simulink model "model2014a"  (R2014a)
settings: Solver=ode4  StartTime=0.0  StopTime=10  FixedStep=0.001  RelTol=1e-3
undefined symbols (not defined in the file): params
libraries: simulink x2
settings Model: Creator=Edo  LastModifiedBy=jelavice
settings DebuggingCC: MergeDetectMultiDrivingBlocksExec=error  FrameProcessingCompatibilityMsg=error

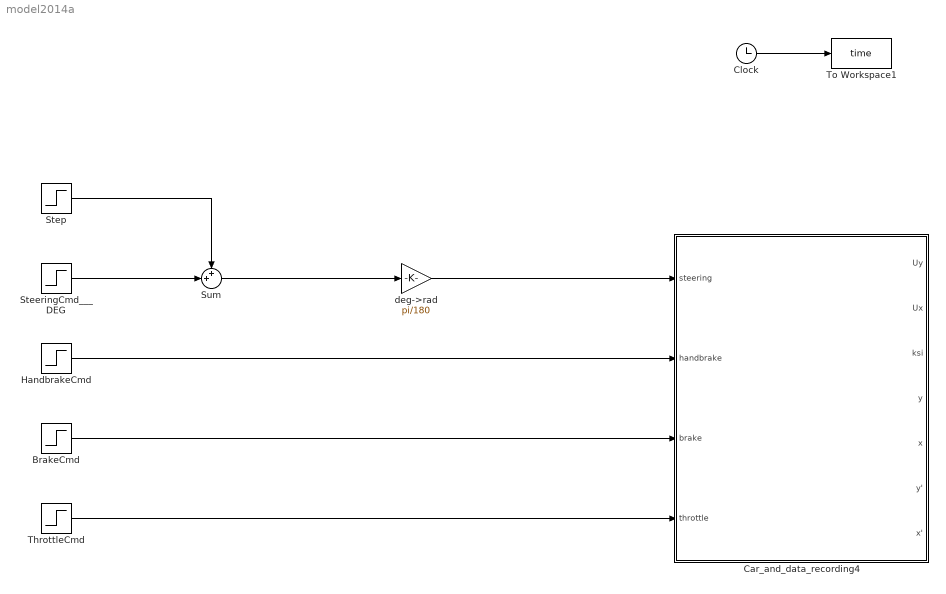
== system model2014a ==
  BrakeCmd : Step  Time=2  After=0  SampleTime=0
  Car_and_data_recording4 : Subsystem
  Clock : Clock
  HandbrakeCmd : Step  Time=3.2  SampleTime=0
  SteeringCmd___DEG : Step  Time=3  After=15  SampleTime=0
  Step : Step  After=0  SampleTime=0
  Sum : Sum  Inputs=++|
  ThrottleCmd : Step  Time=0.1  After=0  SampleTime=0
  To Workspace1 : ToWorkspace  VariableName=time  SampleTime=-1
  deg->rad : Gain  Gain=pi/180
  wires:
  Clock/1 -> To Workspace1/1
  SteeringCmd___DEG/1 -> Sum/2
  Step/1 -> Sum/1
  deg->rad/1 -> Car_and_data_recording4/1(steering)
  BrakeCmd/1 -> Car_and_data_recording4/3(brake)
  HandbrakeCmd/1 -> Car_and_data_recording4/2(handbrake)
  ThrottleCmd/1 -> Car_and_data_recording4/4(throttle)
  Sum/1 -> deg->rad/1

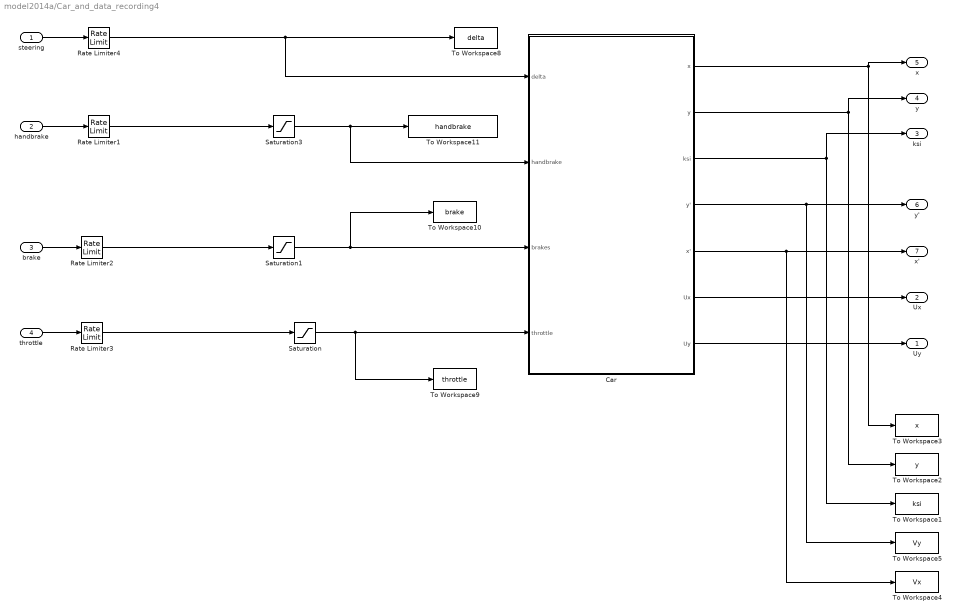
== system model2014a/Car_and_data_recording4 ==
  steering : Inport
  handbrake : Inport  Port=2
  brake : Inport  Port=3
  throttle : Inport  Port=4
  Car : Subsystem
  Rate Limiter1 : RateLimiter  RisingSlewLimit=5  FallingSlewLimit=-5  SampleTimeMode=inherited
  Rate Limiter2 : RateLimiter  RisingSlewLimit=5  FallingSlewLimit=-5  SampleTimeMode=inherited
  Rate Limiter3 : RateLimiter  RisingSlewLimit=5  FallingSlewLimit=-5  SampleTimeMode=inherited
  Rate Limiter4 : RateLimiter  RisingSlewLimit=50*pi/180  FallingSlewLimit=-50*pi/180  SampleTimeMode=inherited
  Saturation : Saturate  UpperLimit=1  LowerLimit=0
  Saturation1 : Saturate  UpperLimit=1  LowerLimit=0
  Saturation3 : Saturate  UpperLimit=1  LowerLimit=0
  To Workspace1 : ToWorkspace  VariableName=ksi  SampleTime=-1
  To Workspace10 : ToWorkspace  VariableName=brake  SampleTime=-1
  To Workspace11 : ToWorkspace  VariableName=handbrake  SampleTime=-1
  To Workspace2 : ToWorkspace  VariableName=y  SampleTime=-1
  To Workspace3 : ToWorkspace  VariableName=x  SampleTime=-1
  To Workspace4 : ToWorkspace  VariableName=Vx  SampleTime=-1
  To Workspace5 : ToWorkspace  VariableName=Vy  SampleTime=-1
  To Workspace8 : ToWorkspace  VariableName=delta  SampleTime=-1
  To Workspace9 : ToWorkspace  VariableName=throttle  SampleTime=-1
  Uy : Outport
  Ux : Outport  Port=2
  ksi : Outport  Port=3
  y : Outport  Port=4
  x : Outport  Port=5
  y' : Outport  Port=6
  x' : Outport  Port=7
  wires:
  Car/3(ksi) -> ksi/1, To Workspace1/1
  Car/2(y) -> y/1, To Workspace2/1
  Car/1(x) -> x/1, To Workspace3/1
  Car/4(y') -> y'/1, To Workspace5/1
  Saturation/1 -> Car/4(throttle), To Workspace9/1
  Saturation1/1 -> Car/3(brakes), To Workspace10/1
  steering/1 -> Rate Limiter4/1
  handbrake/1 -> Rate Limiter1/1
  brake/1 -> Rate Limiter2/1
  Car/5(x') -> x'/1, To Workspace4/1
  Saturation3/1 -> To Workspace11/1, Car/2(handbrake)
  throttle/1 -> Rate Limiter3/1
  Car/6(Ux) -> Ux/1
  Car/7(Uy) -> Uy/1
  Rate Limiter1/1 -> Saturation3/1
  Rate Limiter2/1 -> Saturation1/1
  Rate Limiter3/1 -> Saturation/1
  Rate Limiter4/1 -> To Workspace8/1, Car/1(delta)

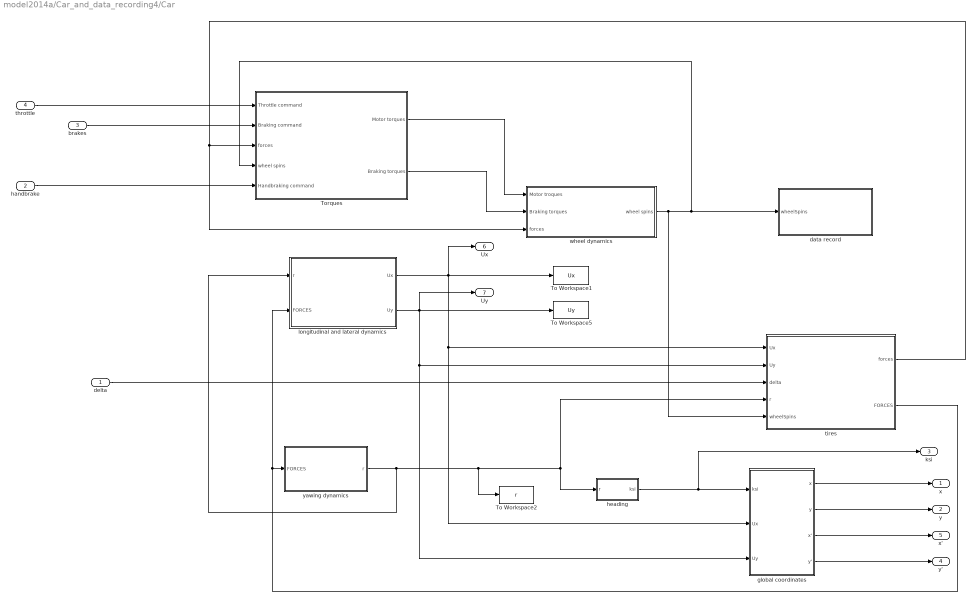
== system model2014a/Car_and_data_recording4/Car ==
  delta : Inport
  handbrake : Inport  Port=2
  brakes : Inport  Port=3
  throttle : Inport  Port=4
  To Workspace1 : ToWorkspace  VariableName=Ux  SampleTime=-1
  To Workspace2 : ToWorkspace  VariableName=r  SampleTime=-1
  To Workspace5 : ToWorkspace  VariableName=Uy  SampleTime=-1
  Torques : Subsystem
  data record : Subsystem
  global coordinates : Subsystem
  "heading " : Subsystem
  longitudinal and lateral dynamics : Subsystem
  tires : Subsystem
  wheel dynamics : Subsystem
  yawing dynamics : Subsystem
  x : Outport
  y : Outport  Port=2
  ksi : Outport  Port=3
  y' : Outport  Port=4
  x' : Outport  Port=5
  Ux : Outport  Port=6
  Uy : Outport  Port=7
  wires:
  Torques/1(Motor torques) -> wheel dynamics/1(Motor troques)
  Torques/2(Braking torques) -> wheel dynamics/2(Braking torques)
  yawing dynamics/1(r) -> longitudinal and lateral dynamics/1(r), To Workspace2/1, tires/4(r), "heading "/1(r)
  longitudinal and lateral dynamics/1(Ux) -> Ux/1, To Workspace1/1, global coordinates/2(Ux), tires/1(Ux)
  longitudinal and lateral dynamics/2(Uy) -> Uy/1, To Workspace5/1, global coordinates/3(Uy), tires/2(Uy)
  global coordinates/1(x) -> x/1
  global coordinates/2(y) -> y/1
  handbrake/1 -> Torques/5(Handbraking command)
  brakes/1 -> Torques/2(Braking command)
  throttle/1 -> Torques/1(Throttle command)
  delta/1 -> tires/3(delta)
  "heading "/1(ksi) -> ksi/1, global coordinates/1(ksi)
  global coordinates/4(y') -> y'/1
  global coordinates/3(x') -> x'/1
  wheel dynamics/1(wheel spins) -> tires/5(wheelSpins), data record/1(wheelSpins), Torques/4(wheel spins)
  tires/2(FORCES) -> yawing dynamics/1(FORCES), longitudinal and lateral dynamics/2(FORCES)
  tires/1(forces) -> wheel dynamics/3(forces), Torques/3(forces)

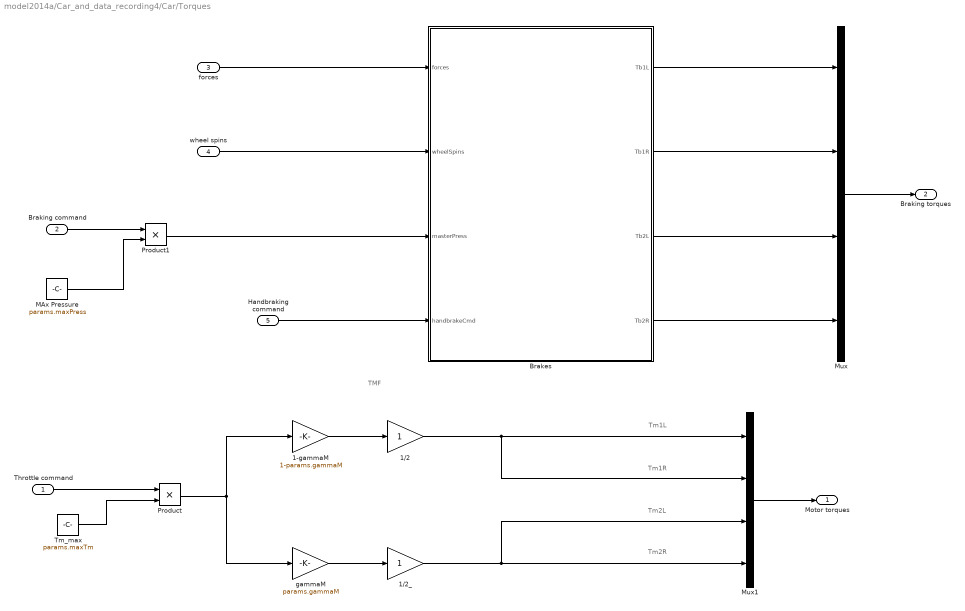
== system model2014a/Car_and_data_recording4/Car/Torques ==
  note: Tm2R
  note: Tm2L
  note: Tm1R
  note: Tm1L
  note: TMF
  Throttle command : Inport
  Braking command : Inport  Port=2
  forces : Inport  Port=3
  wheel spins : Inport  Port=4
  Handbraking command : Inport  Port=5
  1-gammaM : Gain  Gain=1-params.gammaM
  1/2 : Gain
  1/2_ : Gain
  Brakes : MATLAB Function  TreatAsAtomicUnit=on
      settings: PermitHierarchicalResolution=ParametersOnly
  MAx Pressure : Constant  Value=params.maxPress
  Mux : Mux
  Mux1 : Mux
  Product : Product
  Product1 : Product
  Tm_max : Constant  Value=params.maxTm
  gammaM : Gain  Gain=params.gammaM
  Motor torques : Outport
  Braking torques : Outport  Port=2
  wires:
  Throttle command/1 -> Product/1
  Tm_max/1 -> Product/2
  MAx Pressure/1 -> Product1/2
  Braking command/1 -> Product1/1
  Brakes/1(Tb1L) -> Mux/1
  Brakes/2(Tb1R) -> Mux/2
  Mux/1 -> Braking torques/1
  Mux1/1 -> Motor torques/1
  Product/1 -> 1-gammaM/1, gammaM/1
  wheel spins/1 -> Brakes/2(wheelSpins)
  Product1/1 -> Brakes/3(masterPress)
  Handbraking command/1 -> Brakes/4(handbrakeCmd)
  forces/1 -> Brakes/1(forces)
  Brakes/3(Tb2L) -> Mux/3
  Brakes/4(Tb2R) -> Mux/4
  1-gammaM/1 -> 1/2/1
  gammaM/1 -> 1/2_/1
  1/2/1 -> Mux1/2, Mux1/1
  1/2_/1 -> Mux1/4, Mux1/3

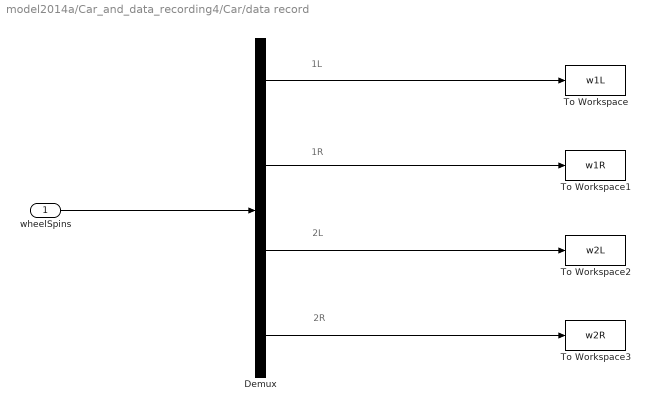
== system model2014a/Car_and_data_recording4/Car/data record ==
  note: 2R
  note: 2L
  note: 1R
  note: 1L
  wheelSpins : Inport
  Demux : Demux
  To Workspace : ToWorkspace  VariableName=w1L  SampleTime=-1
  To Workspace1 : ToWorkspace  VariableName=w1R  SampleTime=-1
  To Workspace2 : ToWorkspace  VariableName=w2L  SampleTime=-1
  To Workspace3 : ToWorkspace  VariableName=w2R  SampleTime=-1
  wires:
  Demux/1 -> To Workspace/1
  Demux/2 -> To Workspace1/1
  Demux/3 -> To Workspace2/1
  Demux/4 -> To Workspace3/1
  wheelSpins/1 -> Demux/1

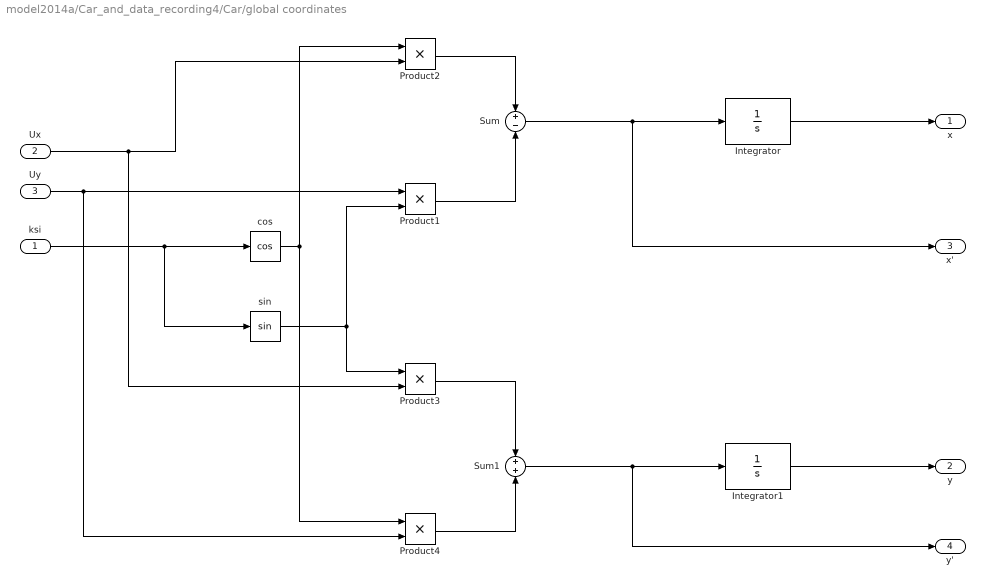
== system model2014a/Car_and_data_recording4/Car/global coordinates ==
  ksi : Inport
  Ux : Inport  Port=2
  Uy : Inport  Port=3
  Integrator : Integrator  InitialCondition=params.x0
  Integrator1 : Integrator  InitialCondition=params.y0
  Product{1..4} (4 alike) : Product
  Sum : Sum  Inputs=+|-
  Sum1 : Sum  Inputs=+|+
  cos : Trigonometry  Operator=cos
  sin : Trigonometry
  x : Outport
  y : Outport  Port=2
  x' : Outport  Port=3
  y' : Outport  Port=4
  wires:
  Integrator/1 -> x/1
  ksi/1 -> sin/1, cos/1
  cos/1 -> Product4/1, Product2/1
  Integrator1/1 -> y/1
  Ux/1 -> Product3/2, Product2/2
  Product2/1 -> Sum/1
  Sum/1 -> x'/1, Integrator/1
  Product1/1 -> Sum/2
  Uy/1 -> Product4/2, Product1/1
  sin/1 -> Product3/1, Product1/2
  Product3/1 -> Sum1/1
  Product4/1 -> Sum1/2
  Sum1/1 -> y'/1, Integrator1/1

== system model2014a/Car_and_data_recording4/Car/heading  ==
  r : Inport
  Integrator : Integrator  InitialCondition=params.ksi0
  ksi : Outport
  wires:
  Integrator/1 -> ksi/1
  r/1 -> Integrator/1

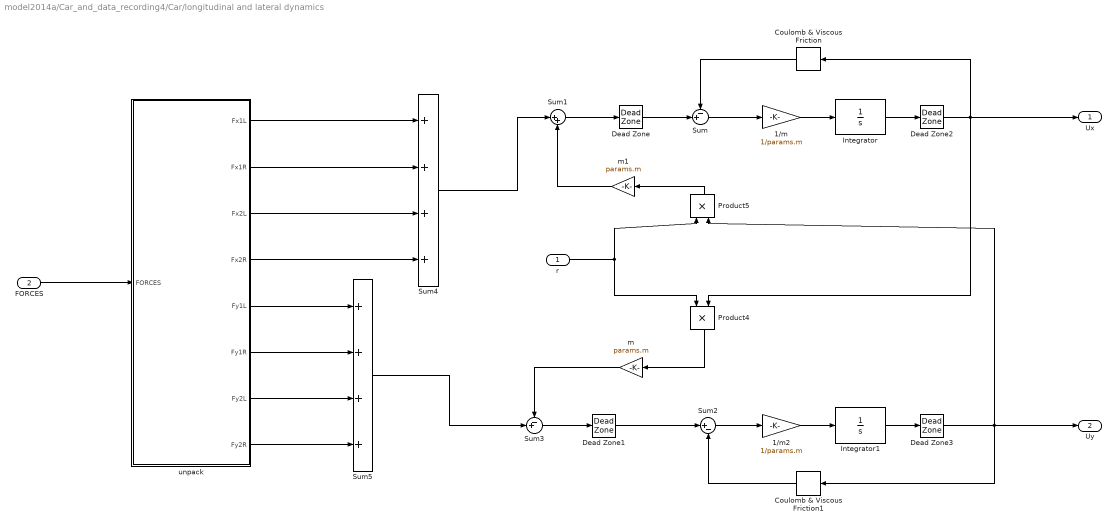
== system model2014a/Car_and_data_recording4/Car/longitudinal and lateral dynamics ==
  r : Inport
  FORCES : Inport  Port=2
  1/m : Gain  Gain=1/params.m
  1/m2 : Gain  Gain=1/params.m
  Coulomb & Viscous Friction : simulink/Discontinuities/Coulomb & Viscous Friction  offset=params.fric  gain=params.b
  Coulomb & Viscous Friction1 : simulink/Discontinuities/Coulomb & Viscous Friction  offset=params.fric*0  gain=params.b*0
  Dead Zone : DeadZone  LowerValue=-params.m*params.g*params.muRoll  UpperValue=params.m*params.g*params.muRoll  SaturateOnIntegerOverflow=on
  Dead Zone1 : DeadZone  LowerValue=-params.m*params.g*params.muRoll  UpperValue=params.m*params.g*params.muRoll  SaturateOnIntegerOverflow=on
  Dead Zone2 : DeadZone  LowerValue=-params.Dz1  UpperValue=params.Dz1  SaturateOnIntegerOverflow=on
  Dead Zone3 : DeadZone  LowerValue=-params.Dz1  UpperValue=params.Dz1  SaturateOnIntegerOverflow=on
  Integrator : Integrator  InitialCondition=params.Ux0
  Integrator1 : Integrator  InitialCondition=params.Uy0
  Product4 : Product
  Product5 : Product
  Sum : Sum  Inputs=-+|
  Sum1 : Sum  Inputs=|++
  Sum2 : Sum  Inputs=|+-
  Sum3 : Sum  Inputs=-+|
  Sum4 : Sum  Inputs=++++
  Sum5 : Sum  Inputs=++++
  m : Gain  Gain=params.m
  m1 : Gain  Gain=params.m
  unpack : Subsystem
  Ux : Outport
  Uy : Outport  Port=2
  wires:
  Sum2/1 -> 1/m2/1
  Product4/1 -> m/1
  r/1 -> Product5/1, Product4/1
  Integrator1/1 -> Dead Zone3/1
  Integrator/1 -> Dead Zone2/1
  Dead Zone1/1 -> Sum2/1
  1/m2/1 -> Integrator1/1
  m/1 -> Sum3/1
  Sum3/1 -> Dead Zone1/1
  Sum5/1 -> Sum3/2
  1/m/1 -> Integrator/1
  Sum4/1 -> Sum1/1
  Sum1/1 -> Dead Zone/1
  Product5/1 -> m1/1
  Dead Zone/1 -> Sum/2
  Sum/1 -> 1/m/1
  Coulomb & Viscous Friction/1 -> Sum/1
  m1/1 -> Sum1/2
  Dead Zone2/1 -> Coulomb & Viscous Friction/1, Ux/1, Product4/2
  Dead Zone3/1 -> Coulomb & Viscous Friction1/1, Uy/1, Product5/2
  FORCES/1 -> unpack/1(FORCES)
  unpack/1(Fx1L) -> Sum4/1
  unpack/2(Fx1R) -> Sum4/2
  unpack/3(Fx2L) -> Sum4/3
  unpack/4(Fx2R) -> Sum4/4
  unpack/5(Fy1L) -> Sum5/1
  unpack/6(Fy1R) -> Sum5/2
  unpack/7(Fy2L) -> Sum5/3
  unpack/8(Fy2R) -> Sum5/4
  Coulomb & Viscous Friction1/1 -> Sum2/2

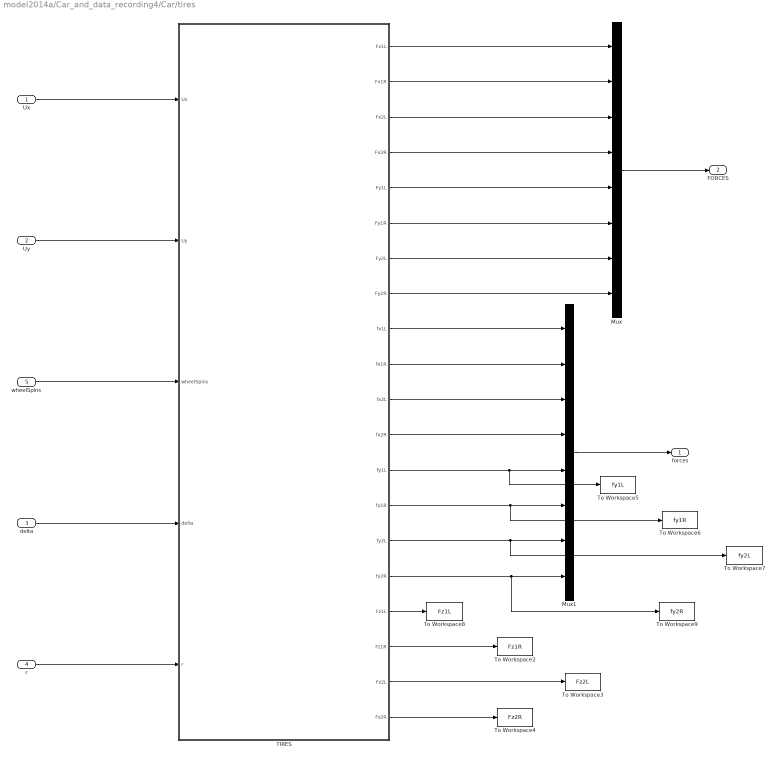
== system model2014a/Car_and_data_recording4/Car/tires ==
  Ux : Inport
  Uy : Inport  Port=2
  delta : Inport  Port=3
  r : Inport  Port=4
  wheelSpins : Inport  Port=5
  Mux : Mux  Inputs=8
  Mux1 : Mux  Inputs=8
  TIRES : MATLAB Function  TreatAsAtomicUnit=on
      settings: PermitHierarchicalResolution=ParametersOnly
  To Workspace2 : ToWorkspace  VariableName=Fz1R  SampleTime=-1
  To Workspace3 : ToWorkspace  VariableName=Fz2L  SampleTime=-1
  To Workspace4 : ToWorkspace  VariableName=Fz2R  SampleTime=-1
  To Workspace5 : ToWorkspace  VariableName=fy1L  SampleTime=-1
  To Workspace6 : ToWorkspace  VariableName=fy1R  SampleTime=-1
  To Workspace7 : ToWorkspace  VariableName=fy2L  SampleTime=-1
  To Workspace8 : ToWorkspace  VariableName=Fz1L  SampleTime=-1
  To Workspace9 : ToWorkspace  VariableName=fy2R  SampleTime=-1
  forces : Outport
  FORCES : Outport  Port=2
  wires:
  Ux/1 -> TIRES/1(Ux)
  Uy/1 -> TIRES/2(Uy)
  delta/1 -> TIRES/4(delta)
  r/1 -> TIRES/5(r)
  Mux/1 -> FORCES/1
  TIRES/1(Fx1L) -> Mux/1
  TIRES/2(Fx1R) -> Mux/2
  TIRES/3(Fx2L) -> Mux/3
  TIRES/4(Fx2R) -> Mux/4
  TIRES/5(Fy1L) -> Mux/5
  TIRES/6(Fy1R) -> Mux/6
  TIRES/7(Fy2L) -> Mux/7
  TIRES/8(Fy2R) -> Mux/8
  wheelSpins/1 -> TIRES/3(wheelSpins)
  TIRES/9(fx1L) -> Mux1/1
  TIRES/14(fy1R) -> To Workspace6/1, Mux1/6
  TIRES/10(fx1R) -> Mux1/2
  TIRES/13(fy1L) -> To Workspace5/1, Mux1/5
  TIRES/11(fx2L) -> Mux1/3
  TIRES/12(fx2R) -> Mux1/4
  TIRES/16(fy2R) -> To Workspace9/1, Mux1/8
  Mux1/1 -> forces/1
  TIRES/17(Fz1L) -> To Workspace8/1
  TIRES/18(Fz1R) -> To Workspace2/1
  TIRES/19(Fz2L) -> To Workspace3/1
  TIRES/20(Fz2R) -> To Workspace4/1
  TIRES/15(fy2L) -> To Workspace7/1, Mux1/7

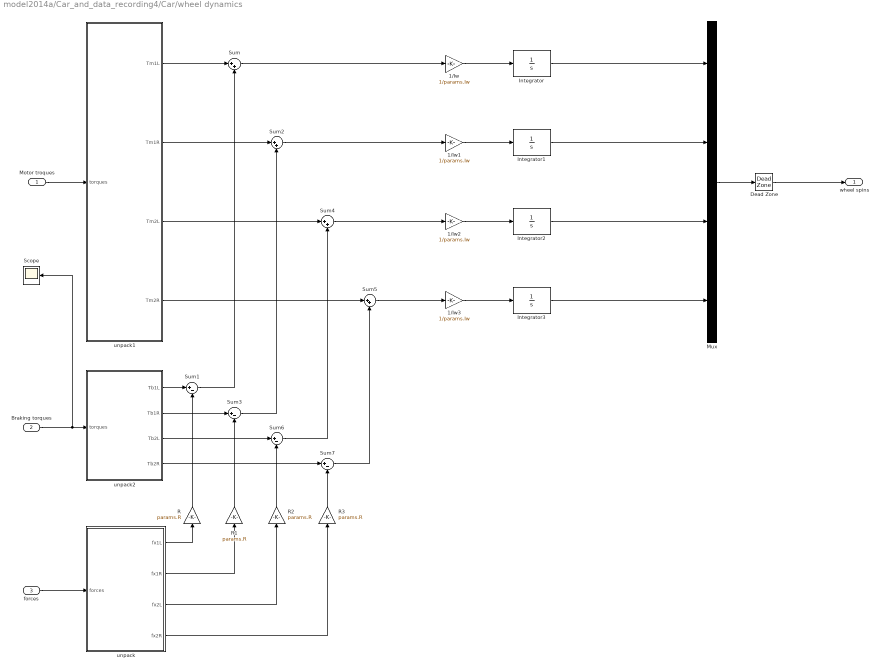
== system model2014a/Car_and_data_recording4/Car/wheel dynamics ==
  Motor troques : Inport
  Braking torques : Inport  Port=2
  forces : Inport  Port=3
  1/Iw{,1..3} (4 alike) : Gain  Gain=1/params.Iw
  Dead Zone : DeadZone  LowerValue=-params.Dz1/params.R  UpperValue=params.Dz1/params.R  SaturateOnIntegerOverflow=on
  Integrator : Integrator  InitialCondition=params.w1L0  LimitOutput=on  LowerSaturationLimit=0
  Integrator1 : Integrator  InitialCondition=params.w1R0  LimitOutput=on  LowerSaturationLimit=0
  Integrator2 : Integrator  InitialCondition=params.w2L0  LimitOutput=on  LowerSaturationLimit=0
  Integrator3 : Integrator  InitialCondition=params.w2R0  LimitOutput=on  LowerSaturationLimit=0
  Mux : Mux
  R{,1..3} (4 alike) : Gain  Gain=params.R
  Scope : Scope
      settings: TimeRange=auto  MaxDataPoints=5000  SaveToWorkspace=off  SaveName=ScopeData  YMin=-10  YMax=10  SampleTime=-1  DataFormat=Array
  Sum{,2,4..5} (4 alike) : Sum  Inputs=|++
  Sum{1,3,6..7} (4 alike) : Sum  Inputs=|+-
  unpack : Subsystem
  unpack1 : Subsystem
  unpack2 : Subsystem
  wheel spins : Outport  PortDimensions=4
  wires:
  1/Iw/1 -> Integrator/1
  1/Iw1/1 -> Integrator1/1
  forces/1 -> unpack/1(forces)
  Motor troques/1 -> unpack1/1(torques)
  Braking torques/1 -> Scope/1, unpack2/1(torques)
  unpack1/1(Tm1L) -> Sum/1
  unpack/1(fx1L) -> R/1
  unpack2/1(Tb1L) -> Sum1/1
  Sum1/1 -> Sum/2
  Sum/1 -> 1/Iw/1
  unpack1/2(Tm1R) -> Sum2/1
  unpack2/2(Tb1R) -> Sum3/1
  unpack/2(fx1R) -> R1/1
  Sum3/1 -> Sum2/2
  Sum2/1 -> 1/Iw1/1
  1/Iw2/1 -> Integrator2/1
  unpack1/3(Tm2L) -> Sum4/1
  Sum4/1 -> 1/Iw2/1
  unpack1/4(Tm2R) -> Sum5/1
  1/Iw3/1 -> Integrator3/1
  Sum5/1 -> 1/Iw3/1
  unpack2/3(Tb2L) -> Sum6/1
  unpack/3(fx2L) -> R2/1
  Sum6/1 -> Sum4/2
  unpack2/4(Tb2R) -> Sum7/1
  unpack/4(fx2R) -> R3/1
  Sum7/1 -> Sum5/2
  R/1 -> Sum1/2
  R1/1 -> Sum3/2
  R2/1 -> Sum6/2
  R3/1 -> Sum7/2
  Mux/1 -> Dead Zone/1
  Integrator/1 -> Mux/1
  Integrator1/1 -> Mux/2
  Integrator2/1 -> Mux/3
  Integrator3/1 -> Mux/4
  Dead Zone/1 -> wheel spins/1

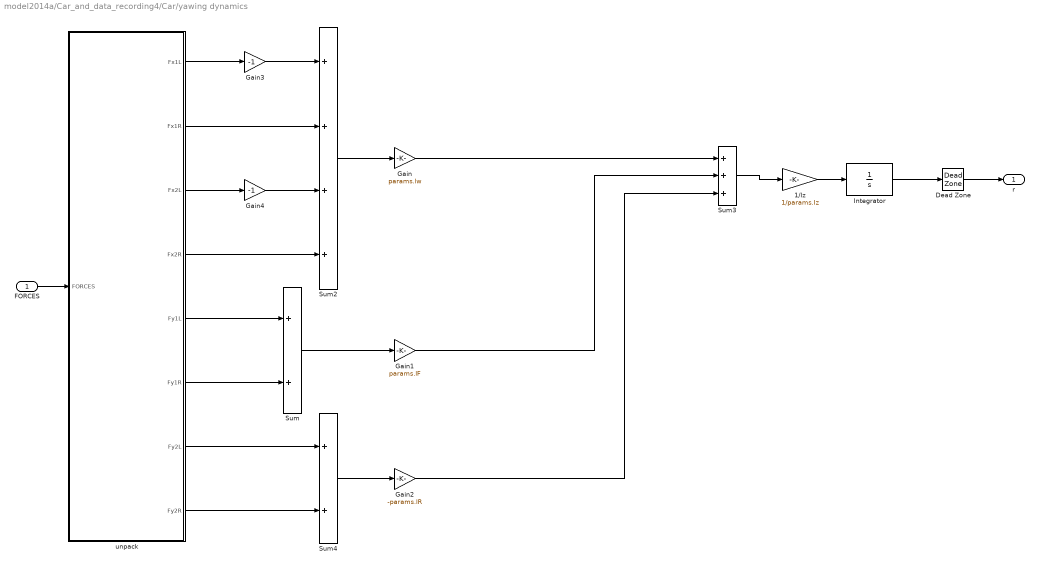
== system model2014a/Car_and_data_recording4/Car/yawing dynamics ==
  FORCES : Inport
  1/Iz : Gain  Gain=1/params.Iz
  Dead Zone : DeadZone  LowerValue=-params.Dz2  UpperValue=params.Dz2  SaturateOnIntegerOverflow=on
  Gain : Gain  Gain=params.lw
  Gain1 : Gain  Gain=params.lF
  Gain2 : Gain  Gain=-params.lR
  Gain3 : Gain  Gain=-1
  Gain4 : Gain  Gain=-1
  Integrator : Integrator  InitialCondition=params.r0
  Sum : Sum
  Sum2 : Sum  Inputs=++++
  Sum3 : Sum  Inputs=+++
  Sum4 : Sum
  unpack : Subsystem
  r : Outport
  wires:
  1/Iz/1 -> Integrator/1
  Sum3/1 -> 1/Iz/1
  Integrator/1 -> Dead Zone/1
  Dead Zone/1 -> r/1
  Sum2/1 -> Gain/1
  Sum4/1 -> Gain2/1
  Sum/1 -> Gain1/1
  unpack/2(Fx1R) -> Sum2/2
  unpack/4(Fx2R) -> Sum2/4
  Gain/1 -> Sum3/1
  Gain1/1 -> Sum3/2
  Gain2/1 -> Sum3/3
  FORCES/1 -> unpack/1(FORCES)
  unpack/1(Fx1L) -> Gain3/1
  unpack/3(Fx2L) -> Gain4/1
  unpack/5(Fy1L) -> Sum/1
  unpack/6(Fy1R) -> Sum/2
  unpack/7(Fy2L) -> Sum4/1
  unpack/8(Fy2R) -> Sum4/2
  Gain4/1 -> Sum2/3
  Gain3/1 -> Sum2/1

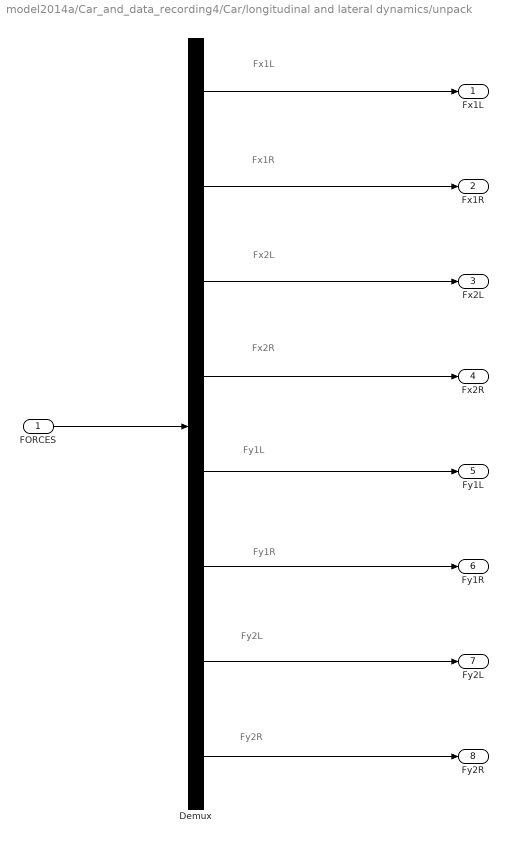
== system model2014a/Car_and_data_recording4/Car/longitudinal and lateral dynamics/unpack ==
  note: Fy2R
  note: Fy2L
  note: Fy1R
  note: Fy1L
  note: Fx2R
  note: Fx2L
  note: Fx1R
  note: Fx1L
  FORCES : Inport
  Demux : Demux  Outputs=8
  Fx1L : Outport
  Fx1R : Outport  Port=2
  Fx2L : Outport  Port=3
  Fx2R : Outport  Port=4
  Fy1L : Outport  Port=5
  Fy1R : Outport  Port=6
  Fy2L : Outport  Port=7
  Fy2R : Outport  Port=8
  wires:
  FORCES/1 -> Demux/1
  Demux/2 -> Fx1R/1
  Demux/4 -> Fx2R/1
  Demux/6 -> Fy1R/1
  Demux/5 -> Fy1L/1
  Demux/1 -> Fx1L/1
  Demux/3 -> Fx2L/1
  Demux/7 -> Fy2L/1
  Demux/8 -> Fy2R/1

== system model2014a/Car_and_data_recording4/Car/wheel dynamics/unpack ==
  note: Fy2R
  note: Fy2L
  note: Fy1R
  note: Fy1L
  note: Fx2R
  note: Fx2L
  note: Fx1R
  note: Fx1L
  forces : Inport
  Demux : Demux  Outputs=8
  fx1L : Outport
  fx1R : Outport  Port=2
  fx2L : Outport  Port=3
  fx2R : Outport  Port=4
  wires:
  forces/1 -> Demux/1
  Demux/1 -> fx1L/1
  Demux/4 -> fx2R/1
  Demux/3 -> fx2L/1
  Demux/2 -> fx1R/1

== system model2014a/Car_and_data_recording4/Car/wheel dynamics/unpack1 ==
  note: Tm2R
  note: Tm2L
  note: Tm1L
  note: Tm1R
  torques : Inport
  Demux1 : Demux
  Tm1L : Outport
  Tm1R : Outport  Port=2
  Tm2L : Outport  Port=3
  Tm2R : Outport  Port=4
  wires:
  torques/1 -> Demux1/1
  Demux1/1 -> Tm1L/1
  Demux1/2 -> Tm1R/1
  Demux1/4 -> Tm2R/1
  Demux1/3 -> Tm2L/1

== system model2014a/Car_and_data_recording4/Car/wheel dynamics/unpack2 ==
  note: Tb2R
  note: Tb2L
  note: Tb1L
  note: Tb1R
  torques : Inport
  Demux1 : Demux
  Tb1L : Outport
  Tb1R : Outport  Port=2
  Tb2L : Outport  Port=3
  Tb2R : Outport  Port=4
  wires:
  torques/1 -> Demux1/1
  Demux1/1 -> Tb1L/1
  Demux1/2 -> Tb1R/1
  Demux1/4 -> Tb2R/1
  Demux1/3 -> Tb2L/1

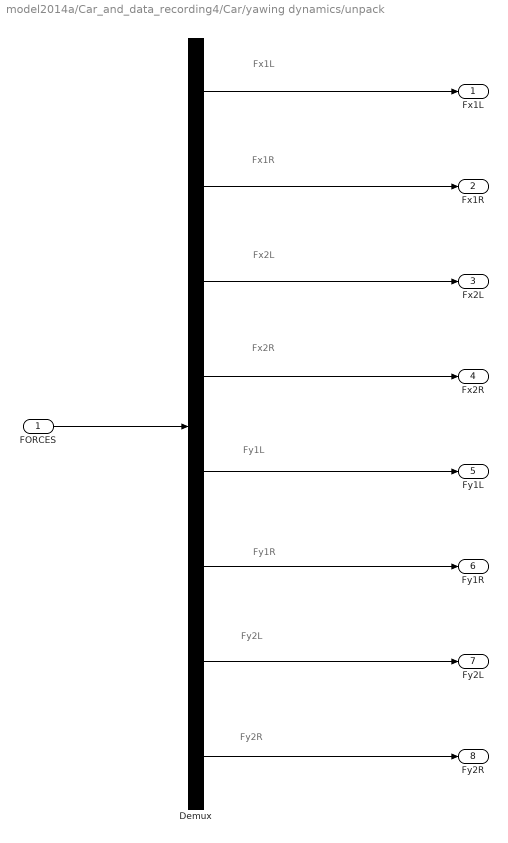
== system model2014a/Car_and_data_recording4/Car/yawing dynamics/unpack ==
  note: Fy2R
  note: Fy2L
  note: Fy1R
  note: Fy1L
  note: Fx2R
  note: Fx2L
  note: Fx1R
  note: Fx1L
  FORCES : Inport
  Demux : Demux  Outputs=8
  Fx1L : Outport
  Fx1R : Outport  Port=2
  Fx2L : Outport  Port=3
  Fx2R : Outport  Port=4
  Fy1L : Outport  Port=5
  Fy1R : Outport  Port=6
  Fy2L : Outport  Port=7
  Fy2R : Outport  Port=8
  wires:
  FORCES/1 -> Demux/1
  Demux/2 -> Fx1R/1
  Demux/4 -> Fx2R/1
  Demux/6 -> Fy1R/1
  Demux/5 -> Fy1L/1
  Demux/1 -> Fx1L/1
  Demux/3 -> Fx2L/1
  Demux/7 -> Fy2L/1
  Demux/8 -> Fy2R/1

== matlab function model2014a/Car_and_data_recording4/Car/Torques/Brakes ==
  data: forces input; Tb1L output; wheelSpins input; params parameter; masterPress input; handbrakeCmd input; Tb1R output; Tb2L output; Tb2R output
function [Tb1L, Tb1R, Tb2L, Tb2R] = brakes(forces,wheelSpins,params, masterPress, handbrakeCmd)
%#codegen

Tb1L = 0;
Tb1R = 0;
Tb2L = 0;
Tb2R = 0;

fx1L = forces(1);
fx1R = forces(2);
fx2L = forces(3);
fx2R = forces(4);

w1L = wheelSpins(1);
w1R = wheelSpins(2);
w2L = wheelSpins(3);
w2R = wheelSpins(4);

pressF = masterPress;
if masterPress <= 1.5
   pressR = masterPress; 
else
   pressR = 0.3 * masterPress + 1.05;
end
    
if masterPress > 0
   
    if w1L ~= 0
        Tb1L = - pressF * params.press2torF*sign(w1L);
    else
        Tb1L = fx1L * params.R;
    end
    
    if w1R ~= 0
        Tb1R = - pressF * params.press2torF*sign(w1R);
    else
        Tb1R = fx1R * params.R;
    end
    
    if w2L ~= 0
        Tb2L = Tb2L - pressR * params.press2torR*sign(w2L);
    else
        Tb2L = fx2L * params.R;
    end
    
    if w2R ~= 0
        Tb2R = Tb2R - pressR * params.press2torR*sign(w2R);
    else
        Tb2R = fx2R * params.R;
    end
end

if handbrakeCmd > 0
   
    if w2L ~= 0
        Tb2L = Tb2L - handbrakeCmd * params.maxThb*sign(w2L);
    else
        Tb2L = fx2L * params.R;
    end   
    
    if w2R ~= 0
        Tb2R = Tb2R - handbrakeCmd * params.maxThb*sign(w2R);
    else
        Tb2R = fx2R * params.R;
    end
end



end

== matlab function model2014a/Car_and_data_recording4/Car/tires/TIRES ==
  data: Ux input; Fx1L output; Uy input; wheelSpins input; delta input; r input; params parameter; Fx1R output; Fx2L output; Fx2R output; Fy1L output; Fy1R output; Fy2L output; Fy2R output; fx1L output; fx1R output; fx2L output; fx2R output; fy1L output; fy1R output; fy2L output; fy2R output; Fz1L output; Fz1R output; Fz2L output; Fz2R output
function [ Fx1L, Fx1R, Fx2L, Fx2R, Fy1L, Fy1R, Fy2L, Fy2R, fx1L, fx1R, fx2L, fx2R, fy1L, fy1R, fy2L, fy2R, Fz1L, Fz1R, Fz2L, Fz2R] = pacejka_model(Ux, Uy, wheelSpins, delta, r, params)
%#codegen

eps = 1e-4;

w1L = wheelSpins(1);
w1R = wheelSpins(2);
w2L = wheelSpins(3);
w2R = wheelSpins(4);

Ux1L = (Ux - r*params.lw)*cos(delta) + (Uy + r*params.lF)*sin(delta);
Uy1L = -(Ux - r*params.lw)*sin(delta) + (Uy + r*params.lF)*cos(delta);

Ux1R = (Ux + r*params.lw)*cos(delta) + (Uy + r*params.lF)*sin(delta);
Uy1R = -(Ux + r*params.lw)*sin(delta) + (Uy + r*params.lF)*cos(delta);

Ux2L = Ux - r*params.lw;
Uy2L = Uy - r*params.lR;

Ux2R = Ux + r*params.lw;
Uy2R = Uy - r*params.lR;


Sx1L = robustDiv2(Ux1L - params.R*w1L, params.R*w1L, eps);
Sy1L = (1+Sx1L) * robustDiv2(Uy1L, Ux1L, eps);

Sx1R = robustDiv2(Ux1R - params.R*w1R, params.R*w1R, eps);
Sy1R = (1+Sx1R) * robustDiv2(Uy1R, Ux1R, eps);

Sx2L = robustDiv2(Ux2L - params.R*w2L, params.R*w2L, eps);
Sy2L = (1+Sx2L) * robustDiv2(Uy2L, Ux2L, eps);

Sx2R = robustDiv2(Ux1R - params.R*w2R, params.R*w2R, eps);
Sy2R = (1+Sx2R) * robustDiv2(Uy2R, Ux2R, eps);



S1L = sqrt( (Sx1L)^2 + (Sy1L)^2 );
S1R = sqrt( (Sx1R)^2 + (Sy1R)^2 );
S2L = sqrt( (Sx2L)^2 + (Sy2L)^2 );
S2R = sqrt( (Sx2R)^2 + (Sy2R)^2 );

mu1L = params.D1*sin(params.C1*atan(params.B1*S1L));
mu1R = params.D1*sin(params.C1*atan(params.B1*S1R));
mu2L = params.D2*sin(params.C2*atan(params.B2*S2L));
mu2R = params.D2*sin(params.C2*atan(params.B2*S2R));

mux1L = - mu1L * robustDiv(Sx1L,S1L,eps);
muy1L = - mu1L * robustDiv(Sy1L,S1L,eps);

mux1R = - mu1R * robustDiv(Sx1R,S1R,eps);
muy1R = - mu1R * robustDiv(Sy1R,S1R,eps);

mux2L = - mu2L * robustDiv(Sx2L,S2L,eps);
muy2L = - mu2L * robustDiv(Sy2L,S2L,eps);

mux2R = - mu2R * robustDiv(Sx2R,S2R,eps);
muy2R = - mu2R * robustDiv(Sy2R,S2R,eps);



C1 = -params.mu*mux1L*params.h*sin(delta);
C2 = -params.mu*muy1L*params.h*cos(delta);
C3 = -params.mu*mux1R*params.h*sin(delta);
C4 = -params.mu*muy1R*params.h*cos(delta);
C5 = -params.mu*muy2L*params.h;
C6 = -params.mu*muy2R*params.h;
% 
K1 = params.mu*mux1L*params.h*cos(delta);
K2 = params.mu*muy1L*params.h*sin(delta);
K3 = params.mu*mux1R*params.h*cos(delta);
K4 = params.mu*muy1R*params.h*sin(delta);
K5 = params.mu*mux2L*params.h;
K6 = params.mu*mux2R*params.h;
% 
A = -params.lw - C1 - C2;
B = params.lw - C3 - C4;
C = -params.lw - C5;
D = params.lw - C6;
E = K1 - K2 - params.lF;
F = K3 - K4 - params.lF;
G = K5 + params.lR;
H = K6 + params.lR;

den = 2*(A*F - E*B - A*G + E*C + B*H - D*F - C*H + D*G);

Fz1L = params.m*params.g*(B*G - C*F + B*H - D*F - C*H + D*G)/den;
Fz1R = - params.m*params.g*(A*G - E*C + A*H - E*D + C*H - D*G)/den;
Fz2L = params.m*params.g*(A*F - E*B + A*H - E*D + B*H - D*F)/den;
Fz2R = params.m*params.g*(A*F - E*B - A*G + E*C - B*G + C*F)/den;


% Fz1L = 0.5* params.m*params.g * params.lR / (2.91);
% Fz1R = 0.5* params.m*params.g * params.lR / (2.91);
% Fz2L = 0.5* params.m*params.g * params.lF / (2.91);
% Fz2R = 0.5* params.m*params.g * params.lF / (2.91);



fx1L = params.mu*Fz1L*mux1L;
fy1L = params.mu*Fz1L*muy1L;

fx1R = params.mu*Fz1R*mux1R;
fy1R = params.mu*Fz1R*muy1R;

fx2L = params.mu*Fz2L*mux2L;
fy2L = params.mu*Fz2L*muy2L;

fx2R = params.mu*Fz2R*mux2R;
fy2R = params.mu*Fz2R*muy2R;


% now change coordinate system

Fx1L = fx1L*cos(delta) - fy1L*sin(delta);
Fy1L = fx1L*sin(delta) + fy1L*cos(delta);

Fx1R = fx1R*cos(delta) - fy1R*sin(delta);
Fy1R = fx1R*sin(delta) + fy1R*cos(delta);

Fx2L = fx2L;
Fy2L = fy2L;

Fx2R = fx2R;
Fy2R = fy2R;

end

function z = robustDiv(num,den, epsilon)

if den == 0 
    if num ~= 0
        z = num/epsilon;
    else
        z = 0; %this is static friction let's say
    end
else
    z = num/den;
end  
      
end

function z = robustDiv2(num,den, epsilon)

if den == 0 
    if abs(num) > epsilon
        z = num/epsilon;
    else
        z = 0; %this is static friction let's say
    end
else
    z = num/den;
end  
        
end
